simulink model "raddrehzahl_filter"  (R2019b)
settings: Solver=FixedStepAuto  StartTime=0.0  StopTime=10.0  RelTol=1e-3
undefined symbols (not defined in the file or in its folder): denom_drehzahl, num_drehzahl
libraries: robotlib x7

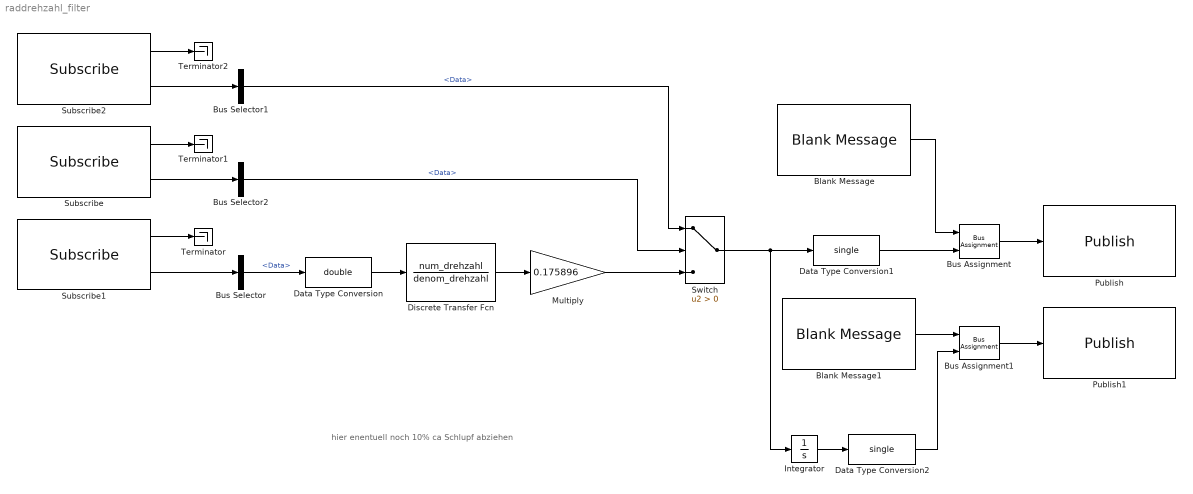
== system raddrehzahl_filter ==
  note: hier enentuell noch 10% ca Schlupf abziehen
  Blank Message : robotlib/Blank Message  messageClass=Message  entityType=std_msgs/Float32  messageType=std_msgs/Float32  SampleTime=inf
  Blank Message1 : robotlib/Blank Message  messageClass=Message  entityType=std_msgs/Float32  messageType=std_msgs/Float32  SampleTime=inf
  Bus Assignment : BusAssignment  AssignedSignals=Data
  Bus Assignment1 : BusAssignment  AssignedSignals=Data
  Bus Selector : BusSelector  OutputSignals=Data
  Bus Selector1 : BusSelector  OutputSignals=Data
  Bus Selector2 : BusSelector  OutputSignals=Data
  Data Type Conversion : DataTypeConversion  OutDataTypeStr=double
  Data Type Conversion1 : DataTypeConversion  OutDataTypeStr=single
  Data Type Conversion2 : DataTypeConversion  OutDataTypeStr=single
  Discrete Transfer Fcn : DiscreteTransferFcn  Numerator=num_drehzahl  Denominator=denom_drehzahl
  Integrator : Integrator
  Multiply : Gain  Gain=0.175896
  Publish : robotlib/Publish  topicSource=Specify your own  topic=/ctl_velocity  messageType=std_msgs/Float32  messageQueueLength=1
  Publish1 : robotlib/Publish  topicSource=Specify your own  topic=/ctl_distance  messageType=std_msgs/Float32  messageQueueLength=1
  Subscribe : robotlib/Subscribe  topicSource=Specify your own  topic=/ctl_withoutSensorValues  messageType=std_msgs/Bool  sampleTime=-1  messageQueueLength=1
  Subscribe1 : robotlib/Subscribe  topicSource=Specify your own  topic=/sns_wheelRpm  messageType=std_msgs/Float32  sampleTime=-1  messageQueueLength=1
  Subscribe2 : robotlib/Subscribe  topicSource=Specify your own  topic=/trj_targetSpeed  messageType=std_msgs/Float32  sampleTime=-1  messageQueueLength=1
  Switch : Switch  Criteria=u2 > Threshold
  Terminator : Terminator
  Terminator1 : Terminator
  Terminator2 : Terminator
  wires:
  Subscribe1/2 -> Bus Selector/1
  Bus Selector/1 -> Data Type Conversion/1  "<Data>"
  Subscribe1/1 -> Terminator/1
  Blank Message/1 -> Bus Assignment/1
  Discrete Transfer Fcn/1 -> Multiply/1
  Bus Assignment/1 -> Publish/1
  Bus Assignment1/1 -> Publish1/1
  Blank Message1/1 -> Bus Assignment1/1
  Integrator/1 -> Data Type Conversion2/1
  Data Type Conversion/1 -> Discrete Transfer Fcn/1
  Data Type Conversion1/1 -> Bus Assignment/2
  Data Type Conversion2/1 -> Bus Assignment1/2
  Subscribe/1 -> Terminator1/1
  Multiply/1 -> Switch/3
  Switch/1 -> Integrator/1, Data Type Conversion1/1
  Subscribe2/1 -> Terminator2/1
  Bus Selector1/1 -> Switch/1  "<Data>"
  Subscribe2/2 -> Bus Selector1/1
  Subscribe/2 -> Bus Selector2/1
  Bus Selector2/1 -> Switch/2  "<Data>"
